simulink model "ep4_2"  (R2023b)
settings: Solver=VariableStepDiscrete  StartTime=0.0  StopTime=50  RelTol=1e-3
settings Model: Creator=86186  LastModifiedBy=86186

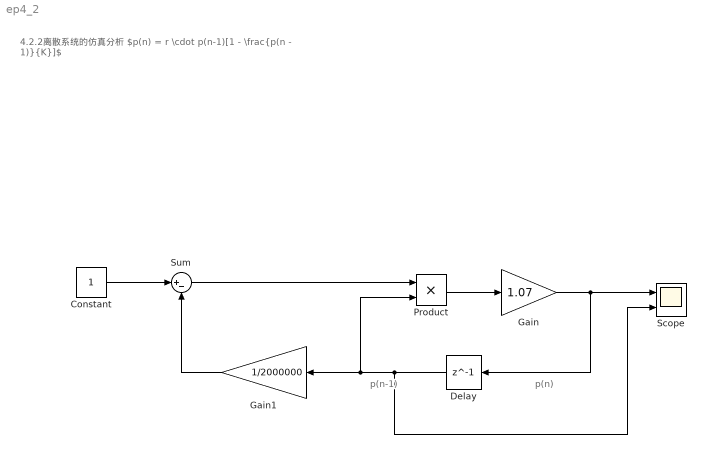
== system ep4_2 ==
  note: 4.2.2离散系统的仿真分析
      | $p(n) = r \cdot p(n-1)[1 - \frac{p(n - 1)}{K}]$
  note: p(n)
  note: p(n-1)
  Constant : Constant
  Delay : Delay  DelayLength=1  InitialCondition=500000
  Gain : Gain  Gain=1.07
  Gain1 : Gain  Gain=1/2000000
  Product : Product
  Scope : Scope  NumInputPorts=2
  Sum : Sum  Inputs=|+-
  wires:
  Gain/1 -> Scope/1, Delay/1
  Delay/1 -> Scope/2, Product/2, Gain1/1
  Gain1/1 -> Sum/2
  Constant/1 -> Sum/1
  Sum/1 -> Product/1
  Product/1 -> Gain/1
